simulink model "WK1L1_DCmachine_sim"  (R2019b)
settings: Solver=VariableStepAuto  StartTime=0.0  StopTime=10.0  RelTol=1e-3
values from neighbouring files (symbols this model uses):
  Bm = 15.1e-4    (= 0.00151)    [LAB_FOCIM_sim.m]    (also in LABprep.m; PMAC_machine.m = 7.59908877318e-07; WK1L1_DCmachine.m = Bm_init + Tmax*(i/10)*0.01; WK2_InductionMachine.m = 0.0337986596081)
  J = 27.6e-3    (= 0.0276)    [LAB_FOCIM_sim.m]    (also in LABprep.m; PMAC_machine.m = 2.55e-08; WK1L1_DCmachine.m = 0.134; WK2_InductionMachine.m = 0.0068)
  k_v = 1.11    [WK1L1_DCmachine.m]
  L_a = 43.8e-3    (= 0.0438)    [WK1L1_DCmachine.m]
  ra = 2.56    [WK1L1_DCmachine.m]
  Va_max = 400    [LABprep.m]    (also in WK1L1_DCmachine.m = Va_max_init*(j/10))
settings Model: Creator=Job  LastModifiedBy=Job
settings DataIOCC: ReturnWorkspaceOutputs=off
settings DebuggingCC: ArithmeticOperatorsInVariantConditions=warning
settings SFSimCC: CustomCodeUndefinedFunction=UseInterfaceOnly

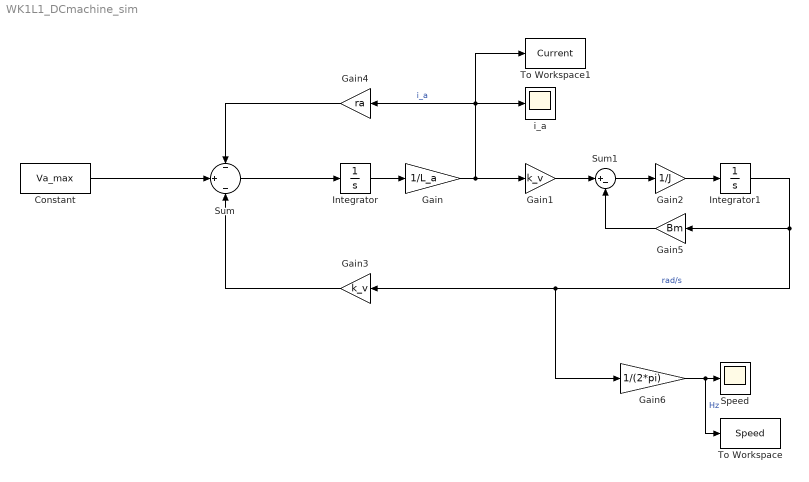
== system WK1L1_DCmachine_sim ==
  Constant : Constant  Value=Va_max
  Gain : Gain  Gain=1/L_a
  Gain1 : Gain  Gain=k_v
  Gain2 : Gain  Gain=1/J
  Gain3 : Gain  Gain=k_v
  Gain4 : Gain  Gain=ra
  Gain5 : Gain  Gain=Bm
  Gain6 : Gain  Gain=1/(2*pi)
  Integrator : Integrator
  Integrator1 : Integrator
  Speed : Scope
  Sum : Sum  Inputs=-|+|-
  Sum1 : Sum  Inputs=|+-
  To Workspace : ToWorkspace  VariableName=Speed  SampleTime=-1
  To Workspace1 : ToWorkspace  VariableName=Current  SampleTime=-1
  i_a : Scope
  wires:
  Constant/1 -> Sum/2
  Sum/1 -> Integrator/1
  Integrator/1 -> Gain/1
  Gain/1 -> To Workspace1/1, Gain4/1, i_a/1, Gain1/1  "i_a"
  Gain1/1 -> Sum1/1
  Sum1/1 -> Gain2/1
  Gain2/1 -> Integrator1/1
  Gain4/1 -> Sum/1
  Gain3/1 -> Sum/3
  Integrator1/1 -> Gain5/1, Gain6/1, Gain3/1  "rad/s"
  Gain5/1 -> Sum1/2
  Gain6/1 -> To Workspace/1, Speed/1  "Hz"
